simulink model "MCP_phase3_compensator_full"  (R2020a)
settings: Solver=VariableStepAuto  StartTime=0.0  StopTime=1500  RelTol=1e-3
values from neighbouring files (symbols this model uses):
  h1_eq = 11.4    [Four_Tank.m]    (also in Four_Tank_phase3_LQR.m; Four_Tank_phase3_nonlinear.m; MCP_phase3_observers.m)
  h2_eq = 11.6    [Four_Tank.m]    (also in Four_Tank_phase3_LQR.m; Four_Tank_phase3_nonlinear.m; MCP_phase3_observers.m)
  h3_eq = 5.3    [Four_Tank.m]    (also in Four_Tank_phase3_LQR.m; Four_Tank_phase3_nonlinear.m = real(double(answer.h3)); MCP_phase3_observers.m)
  h4_eq = 4    [Four_Tank.m]    (also in Four_Tank_phase3_LQR.m; Four_Tank_phase3_nonlinear.m = real(double(answer.h4)); MCP_phase3_observers.m)
  v1_eq = 0.5    [Four_Tank.m]    (also in Four_Tank_phase3_LQR.m; Four_Tank_phase3_nonlinear.m = real(double(answer.v1)); MCP_phase3_observers.m)
  v2_eq = 0.5    [Four_Tank.m]    (also in Four_Tank_phase3_LQR.m; Four_Tank_phase3_nonlinear.m = real(double(answer.v2)); MCP_phase3_observers.m)
settings Model: Creator=rafiee  LastModifiedBy=Lenovo
settings DataIOCC: ReturnWorkspaceOutputs=off
settings DebuggingCC: ArithmeticOperatorsInVariantConditions=warning
settings SFSimCC: SimUseLocalCustomCode=off  CustomCodeUndefinedFunction=UseInterfaceOnly
settings RTWCC: RTWUseLocalCustomCode=off
settings CodeAppCC: StateflowObjectComments=on

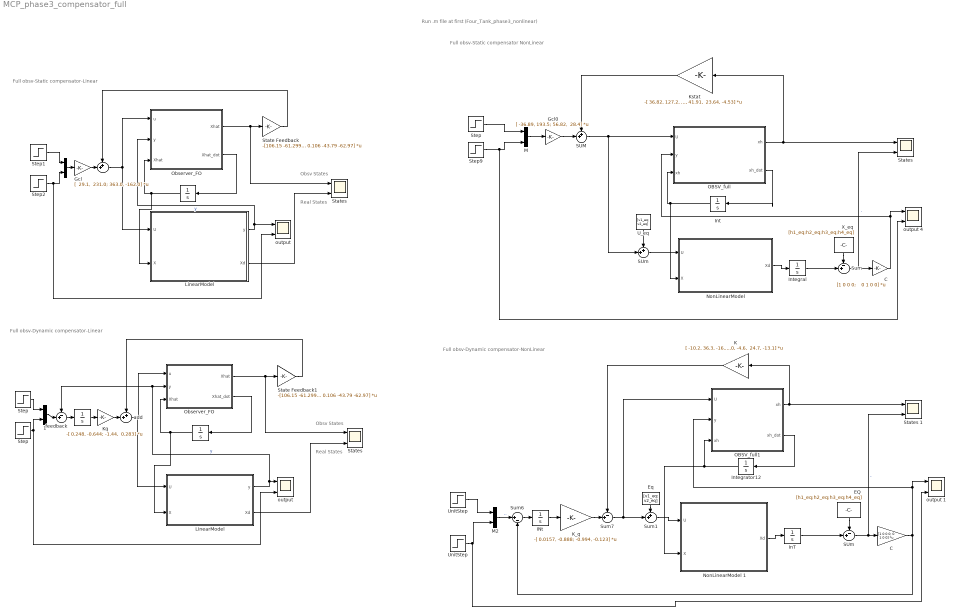
== system MCP_phase3_compensator_full ==
  note: Full obsv-Dynamic compensator-NonLinear
  note: Run .m file at first (Four_Tank_phase3_nonlinear)
  note: Real States
  note: Obsv States
  note: Full obsv-Static compensator-Linear
  note: Real States
  note: Full obsv-Dynamic compensator-Linear
  note: Obsv States
  note: Full obsv-Static compensator NonLinear
  "  " : Integrator  InitialCondition=[0;0;0;0;0;0]
  "   " : Concatenate
  "     " : Sum  Inputs=++|
  "           " : Integrator
  "                      " : Integrator  InitialCondition=[0;0;0;0;0;0]
  "   1" : Concatenate
  " C " : Gain  Gain=|  Multiplication=Matrix(K*u)
      | [1 0 0 0;
      |    0 1 0 0]
  " States " : Scope  NumInputPorts=2
  " States 1" : Scope  NumInputPorts=2
  " Step" : Step  SampleTime=0
  " Sum" : Sum  Inputs=-+|
  " add" : Sum  Inputs=++|
  " feedback" : Sum  Inputs=-+|
  " output " : Scope  NumInputPorts=2
  "C " : Gain  Gain=|  Multiplication=Matrix(K*u)
      | [1 0 0 0;
      |    0 1 0 0]
  EQ : Constant  Value=[h1_eq;h2_eq;h3_eq;h4_eq]
  Eq : Constant  Value=[v1_eq; v2_eq]
  Gcl : Gain  Gain="[  29.1,  231.0; 363.0, -162.0]"  Multiplication=Matrix(K*u)
  Gcl0 : Gain  Gain="[ -36.89, 193.5; 56.82,  28.4]"  Multiplication=Matrix(K*u)
  INt : Integrator
  InT : Integrator  InitialCondition=[h1_eq; h2_eq; h3_eq; h4_eq]
  Int : Integrator  InitialCondition=[0;0;0;0]
  Integral : Integrator  InitialCondition=[h1_eq; h2_eq; h3_eq; h4_eq]
  Integrator12 : Integrator  InitialCondition=[0;0;0;0]
  K : Gain  Gain="[ -10.2, 36.3, -16.5,  24.5; 41.0, -4.6,  24.7, -13.1]"  Multiplication=Matrix(K*u)
  "K_q " : Gain  Gain=-[ 0.0157, -0.888; -0.994, -0.123]  Multiplication=Matrix(K*u)
  Kq : Gain  Gain="-[ 0.248, -0.644; -1.44,  0.283]"  Multiplication=Matrix(K*u)
  Kstat : Gain  Gain="-[ 36.82, 127.2, -58.99, 57.97; 31.33, 41.91,  23.64, -4.53]"  Multiplication=Matrix(K*u)
  LinearModel : MATLAB Function  TreatAsAtomicUnit=on
  "LinearModel " : MATLAB Function  TreatAsAtomicUnit=on
  M : Concatenate
  M2 : Concatenate
  "NonLinearModel " : MATLAB Function  TreatAsAtomicUnit=on
  NonLinearModel 1 : MATLAB Function  TreatAsAtomicUnit=on
  OBSV_full : MATLAB Function  TreatAsAtomicUnit=on
  OBSV_full1 : MATLAB Function  TreatAsAtomicUnit=on
  Observer_FO : MATLAB Function  TreatAsAtomicUnit=on
  "Observer_FO " : MATLAB Function  TreatAsAtomicUnit=on
  SUM : Sum  Inputs=++|
  SUm : Sum  Inputs=++|
  "SUm " : Sum  Inputs=-+|
  State Feedback : Gain  Gain=-[106.15 -61.299 0.111 0.986 160.72 57.96; 169.55 189.92 1.35 0.106 -43.79 -62.97]  Multiplication=Matrix(K*u)
  State Feedback1 : Gain  Gain=-[106.15 -61.299 0.111 0.986 160.72 57.96; 169.55 189.92 1.35 0.106 -43.79 -62.97]  Multiplication=Matrix(K*u)
  States : Scope  NumInputPorts=2
  "States " : Scope  NumInputPorts=2
  Step{,1..2,9} (4 alike) : Step  SampleTime=0
  "Step " : Step  SampleTime=0
  Sum1 : Sum  Inputs=++|
  Sum6 : Sum  Inputs=|+-
  Sum7 : Sum  Inputs=-+|
  U_eq : Constant  Value=[v1_eq; v2_eq]
  UnitStep : Step  SampleTime=0
  "UnitStep " : Step  SampleTime=0
  X_eq : Constant  Value=[h1_eq;h2_eq;h3_eq;h4_eq]
  "output " : Scope  NumInputPorts=2
  output 1 : Scope  NumInputPorts=2
  output 4 : Scope  NumInputPorts=2
  wires:
  LinearModel/1(y) -> Observer_FO/2(y), "output "/1  "y"
  State Feedback/1 -> "     "/1
  Observer_FO/2(Xhat_dot) -> "  "/1
  Gcl/1 -> "     "/2
  Step1/1 -> "   "/1
  "   "/1 -> Gcl/1
  "     "/1 -> LinearModel/1(U), Observer_FO/1(u)
  LinearModel/2(Xd) -> States/2
  Step2/1 -> "output "/2, "   "/2
  Observer_FO/1(Xhat) -> States/1, State Feedback/1
  "  "/1 -> LinearModel/2(X), Observer_FO/3("Xhat ")
  " feedback"/1 -> "           "/1
  "           "/1 -> Kq/1
  "   1"/1 -> " feedback"/2
  "Observer_FO "/2(Xhat_dot) -> "                      "/1
  "Observer_FO "/1(Xhat) -> "States "/1, State Feedback1/1
  Kq/1 -> " add"/2
  "                      "/1 -> "LinearModel "/2(X), "Observer_FO "/3("Xhat ")
  "LinearModel "/2(Xd) -> "States "/2
  State Feedback1/1 -> " add"/1
  " add"/1 -> "LinearModel "/1(U), "Observer_FO "/1(u)
  " Step"/1 -> "   1"/2, " output "/2
  "LinearModel "/1(y) -> "Observer_FO "/2(y), " feedback"/1, " output "/1  "y"
  "Step "/1 -> "   1"/1
  "C "/1 -> output 4/1, OBSV_full/2(y)
  Gcl0/1 -> SUM/2
  OBSV_full/2(xh_dot) -> Int/1
  OBSV_full/1(xh) -> " States "/1, Kstat/1
  Step/1 -> M/1
  Int/1 -> "NonLinearModel "/2(X), OBSV_full/3("xh ")
  Kstat/1 -> SUM/1
  SUM/1 -> OBSV_full/1(U), SUm/2
  M/1 -> Gcl0/1
  "NonLinearModel "/1(Xd) -> Integral/1
  SUm/1 -> "NonLinearModel "/1(U)
  " Sum"/1 -> " States "/2, "C "/1  "."
  X_eq/1 -> " Sum"/1
  Step9/1 -> output 4/2, M/2
  Integral/1 -> " Sum"/2
  U_eq/1 -> SUm/1
  "UnitStep "/1 -> output 1/2, M2/2
  " C "/1 -> Sum6/2, output 1/1, OBSV_full1/2(y)
  "SUm "/1 -> " States 1"/2, " C "/1  ","
  K/1 -> Sum7/1
  Integrator12/1 -> NonLinearModel 1/2(X), OBSV_full1/3("xh ")
  Eq/1 -> Sum1/1
  Sum7/1 -> Sum1/2, OBSV_full1/1(U)
  OBSV_full1/2(xh_dot) -> Integrator12/1
  OBSV_full1/1(xh) -> " States 1"/1, K/1
  INt/1 -> "K_q "/1
  Sum6/1 -> INt/1
  NonLinearModel 1/1(Xd) -> InT/1
  "K_q "/1 -> Sum7/2
  InT/1 -> "SUm "/2
  UnitStep/1 -> M2/1
  Sum1/1 -> NonLinearModel 1/1(U)
  EQ/1 -> "SUm "/1
  M2/1 -> Sum6/1  ".."

== matlab function MCP_phase3_compensator_full/Observer_FO ==
  data: Xhat output; u input; Xhat_dot output; y input; Xhat input
function [Xhat, Xhat_dot]= observer_FO(u, y, Xhat)

A = [ -0.0189,  0.029,      0, 0.00306,       0,       0;
       0, -0.029, 0.0065,       0,       0,       0;
       0,      0, -0.476,       0,       0,       0;
       0,      0,      0,    -0.5,       0,       0;
       0,      0, 0.0035,       0, -0.0191,  0.0349;
       0,      0,      0, 0.00714,       0, -0.0349];

B =[0,     0;
   0,     0;
   0, 0.476;
   0.5,     0;
   0,     0;
   0,     0];

C = [1.0, 0, 0, 0, 0, 0;
     0, 0, 0, 0, 1.0, 0];
 
L = [0.367, -0.0766;
      0.77,  -0.525;
    0.257,   -1.66;
 -0.00453,  0.0113;
  -0.0573,   0.655;
   -0.323,    2.12];

Xhat_dot = A*Xhat + B*u + L*(y - C*Xhat);

== matlab function MCP_phase3_compensator_full/LinearModel  ==
  data: y output; U input; X input; Xd output
function [y, Xd]  = linear_plant(U, X)

A = [ -0.0189,  0.029,      0, 0.00306,       0,       0;
       0, -0.029, 0.0065,       0,       0,       0;
       0,      0, -0.476,       0,       0,       0;
       0,      0,      0,    -0.5,       0,       0;
       0,      0, 0.0035,       0, -0.0191,  0.0349;
       0,      0,      0, 0.00714,       0, -0.0349];

B =[0,     0;
   0,     0;
   0, 0.476;
   0.5,     0;
   0,     0;
   0,     0];

C = [1.0, 0, 0, 0, 0, 0;
     0, 0, 0, 0, 1.0, 0];
Xd = A * X + B * U; 
y = C*X;

== matlab function MCP_phase3_compensator_full/LinearModel ==
  data: y output; U input; X input; Xd output
function [y, Xd]  = linear_plant(U, X)

A = [ -0.0189,  0.029,      0, 0.00306,       0,       0;
       0, -0.029, 0.0065,       0,       0,       0;
       0,      0, -0.476,       0,       0,       0;
       0,      0,      0,    -0.5,       0,       0;
       0,      0, 0.0035,       0, -0.0191,  0.0349;
       0,      0,      0, 0.00714,       0, -0.0349];

B =[0,     0;
   0,     0;
   0, 0.476;
   0.5,     0;
   0,     0;
   0,     0];

C = [1.0, 0, 0, 0, 0, 0;
     0, 0, 0, 0, 1.0, 0];
Xd = A * X + B * U; 
y = C*X;

== matlab function MCP_phase3_compensator_full/Observer_FO  ==
  data: Xhat output; u input; Xhat_dot output; y input; Xhat input
function [Xhat, Xhat_dot]= observer_FO(u, y, Xhat)

A = [ -0.0189,  0.029,      0, 0.00306,       0,       0;
       0, -0.029, 0.0065,       0,       0,       0;
       0,      0, -0.476,       0,       0,       0;
       0,      0,      0,    -0.5,       0,       0;
       0,      0, 0.0035,       0, -0.0191,  0.0349;
       0,      0,      0, 0.00714,       0, -0.0349];

B =[0,     0;
   0,     0;
   0, 0.476;
   0.5,     0;
   0,     0;
   0,     0];

C = [1.0, 0, 0, 0, 0, 0;
     0, 0, 0, 0, 1.0, 0];
 
L = [0.367, -0.0766;
      0.77,  -0.525;
    0.257,   -1.66;
 -0.00453,  0.0113;
  -0.0573,   0.655;
   -0.323,    2.12];

Xhat_dot = A*Xhat + B*u + L*(y - C*Xhat);

== matlab function MCP_phase3_compensator_full/NonLinearModel 1 ==
  data: U input; Xd output; X input
function Xd = NonlinearModel(U, X)

A = [730 730 730 730];
a = [2.10 2.14 2.2 2.3];
g = 981;
y = [0.3 0.35];
k = [7.45 7.30];

v1 = U(1);
v2 = U(2);

h1 = X(1);
h2 = X(2);
h3 = X(3);
h4 = X(4);

h1_d = -a(1)/A(1)*sqrt(2*g*h1)+a(3)/A(1)*sqrt(2*g*h3)+y(1)*k(1)/A(1)*v1;
h2_d = -a(2)/A(2)*sqrt(2*g*h2)+a(4)/A(2)*sqrt(2*g*h4)+y(2)*k(2)/A(2)*v2;
h3_d = -a(3)/A(3)*sqrt(2*g*h3)+(1 - y(2))*k(2)/A(3)*v2;
h4_d = -a(4)/A(4)*sqrt(2*g*h4)+(1 - y(1))*k(1)/A(4)*v1;

Xd = [h1_d;h2_d;h3_d;h4_d];

== matlab function MCP_phase3_compensator_full/OBSV_full1 ==
  data: xh output; U input; xh_dot output; y input; xh input
function [xh, xh_dot] = Obsv_Full(U, y ,xh)

A = [ -0.01887,        0,  0.02899,        0;
         0, -0.01906,        0,  0.03489;
        0,        0, -0.02899,        0;
        0,        0,        0, -0.03489];


    B = [ 0.003062,      0;
        0, 0.0035;
        0, 0.0065;
 0.007144,      0];
 
C = [1 0 0 0;
   0 1 0 0];

L = [ 0.8521,     0;
      0, 0.446;
  6.027,     0;
      0, 1.255];
   
xh_dot = A*xh+B*U+L*(y-C*xh);

== matlab function MCP_phase3_compensator_full/NonLinearModel  ==
  data: U input; Xd output; X input
function Xd = NonlinearModel(U, X)

A = [730 730 730 730];
a = [2.10 2.14 2.2 2.3];
g = 981;
y = [0.3 0.35];
k = [7.45 7.30];

v1 = U(1);
v2 = U(2);

h1 = X(1);
h2 = X(2);
h3 = X(3);
h4 = X(4);

h1_d = -a(1)/A(1)*sqrt(2*g*h1)+a(3)/A(1)*sqrt(2*g*h3)+y(1)*k(1)/A(1)*v1;
h2_d = -a(2)/A(2)*sqrt(2*g*h2)+a(4)/A(2)*sqrt(2*g*h4)+y(2)*k(2)/A(2)*v2;
h3_d = -a(3)/A(3)*sqrt(2*g*h3)+(1 - y(2))*k(2)/A(3)*v2;
h4_d = -a(4)/A(4)*sqrt(2*g*h4)+(1 - y(1))*k(1)/A(4)*v1;

Xd = [h1_d;h2_d;h3_d;h4_d];

== matlab function MCP_phase3_compensator_full/OBSV_full ==
  data: xh output; U input; xh_dot output; y input; xh input
function [xh, xh_dot] = Obsv_Full(U, y ,xh)

A = [ -0.01887,        0,  0.02899,        0;
         0, -0.01906,        0,  0.03489;
        0,        0, -0.02899,        0;
        0,        0,        0, -0.03489];


    B = [ 0.003062,      0;
        0, 0.0035;
        0, 0.0065;
 0.007144,      0];
 
C = [1 0 0 0;
   0 1 0 0];

L = [ 0.8521,     0;
      0, 0.446;
  6.027,     0;
      0, 1.255];
   
xh_dot = A*xh+B*U+L*(y-C*xh);
